simulink model "LLIMTest"  (R2020a)
settings: Solver=VariableStepAuto  StartTime=0.0  StopTime=inf  RelTol=1e-3  EnableMultiTasking=on
libraries: simulink x2, dspsigops x1, realtime_pacer_lib x1
settings Model: Creator=tbria  LastModifiedBy=Harjot
settings OptimizationCC: LifeSpan=inf
settings DebuggingCC: SFUnexpectedBacktrackingDiag=warning  SFNoUnconditionalDefaultTransitionDiag=warning  SFExecutionAtInitializationDiag=none  ArithmeticOperatorsInVariantConditions=warning
settings SFSimCC: SimUseLocalCustomCode=off  CustomCodeUndefinedFunction=UseInterfaceOnly
settings RTWCC: RTWUseLocalCustomCode=off
settings CodeAppCC: StateflowObjectComments=on
settings GRTTargetCC: TargetLangStandard=C89/C90 (ANSI)
settings ConfigComp: CovMetricSettings=dw  CovHtmlReporting=on  CovSaveCumulativeToWorkspaceVar=on  CovSaveSingleToWorkspaceVar=on  CovExternalEMLEnable=off

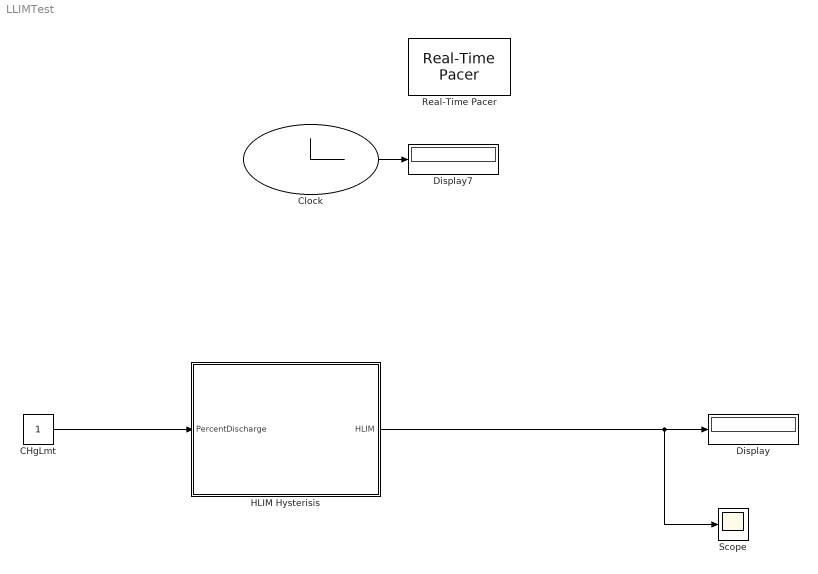
== system LLIMTest ==
  CHgLmt : Constant
  Clock : Clock
  Display : Display
  Display7 : Display
  HLIM Hysterisis : Subsystem
  Real-Time Pacer : realtime_pacer_lib/Real-Time Pacer  simTimePerRealTime=1
      settings: SourceProductName=Real-Time Pacer
  Scope : Scope
  wires:
  Clock/1 -> Display7/1
  HLIM Hysterisis/1(HLIM) -> Scope/1, Display/1
  CHgLmt/1 -> HLIM Hysterisis/1(PercentDischarge)

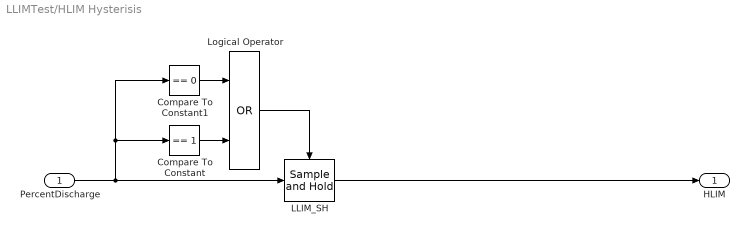
== system LLIMTest/HLIM Hysterisis ==
  PercentDischarge : Inport
  Compare To Constant : simulink/Logic and Bit Operations/Compare To Constant  relop===  const=1  OutDataTypeStr=boolean
  Compare To Constant1 : simulink/Logic and Bit Operations/Compare To Constant  relop===  const=0  OutDataTypeStr=boolean
  LLIM_SH : dspsigops/Sample and Hold  trig=Rising edge  initCond=1  latchinput=off
  Logical Operator : Logic  Operator=OR  AllPortsSameDT=off  OutDataTypeStr=boolean
  HLIM : Outport  VectorParamsAs1DForOutWhenUnconnected=off
  wires:
  Compare To Constant1/1 -> Logical Operator/1
  Compare To Constant/1 -> Logical Operator/2
  Logical Operator/1 -> LLIM_SH/Trigger
  LLIM_SH/1 -> HLIM/1
  PercentDischarge/1 -> Compare To Constant1/1, Compare To Constant/1, LLIM_SH/1
